simulink model "ZPTEC_state_feedback"  (R2020b)
settings: Solver=FixedStepAuto  StartTime=0.0  StopTime=1  FixedStep=0.002  RelTol=1e-3  EnableMultiTasking=on
values from neighbouring files (symbols this model uses):
  A = [0 1 ... (first row only)    [TestDIST_EFFECT_DCmotor_zp(1).m]    (also in TestDIST_EFFECT_DCmotor_zp.m; lqr_DOB_2_5.mat = [0  1; 0  0]; lqr_DOB_5.mat = [0  1; 0  0]; lqr_DOB_8.mat = [0  1; 0  0])
  B = [0; Kt/Rm/Jt]    [TestDIST_EFFECT_DCmotor_zp(1).m]    (also in TestDIST_EFFECT_DCmotor_zp.m; lqr_DOB_2_5.mat = [0 239.250934036]; lqr_DOB_5.mat = [0 239.250934036]; lqr_DOB_8.mat = [0 239.250934036])
  d = [1 -1.75526480336 0.782027160212]    [lqr_DOB_2_5.mat]    (also in lqr_DOB_5.mat; lqr_DOB_8.mat; lqr_noDOB_10.mat = [1 -1.7546251878 0.781376862182]; lqr_noDOB_2_5.mat = [1 -1.7546251878 0.781376862182])
  K = KK    [TestDIST_EFFECT_DCmotor_zp.m]    (also in lqr_DOB_2_5.mat = [27.9647466006 0.483496818901]; lqr_DOB_5.mat = [27.9647466006 0.483496818901]; lqr_DOB_8.mat = [27.9647466006 0.483496818901]; lqr_noDOB_10.mat = [28.2374499722 0.447372514694])
  n = n(2:3)    [TestDIST_EFFECT_DCmotor_zp(1).m]    (also in TestDIST_EFFECT_DCmotor_zp.m; lqr_DOB_2_5.mat = [0.0133811834885 0.0133811834885]; lqr_DOB_5.mat = [0.0133811834885 0.0133811834885]; lqr_DOB_8.mat = [0.0133811834885 0.0133811834885])
settings Model: Creator=oboe  LastModifiedBy=Lab-Mec
settings DataIOCC: LimitDataPoints=on  SaveFormat=Array  ReturnWorkspaceOutputs=off
settings OptimizationCC: LifeSpan=inf
settings DebuggingCC: SolverPrmCheckMsg=warning  SFUnexpectedBacktrackingDiag=warning  SFNoUnconditionalDefaultTransitionDiag=warning  SFExecutionAtInitializationDiag=none  ArithmeticOperatorsInVariantConditions=warning
settings HardwareCC: ProdBitPerPointer=32  ProdBitPerSizeT=32  ProdBitPerPtrDiffT=32  ProdLargestAtomicFloat=None  ProdIntDivRoundTo=Undefined  ProdEndianess=Unspecified  ProdWordSize=32  ProdHWDeviceType=32-bit Generic
settings ModelReferenceCC: PropagateSignalLabelsOutOfModel=off
settings SFSimCC: SimUseLocalCustomCode=off  CustomCodeUndefinedFunction=UseInterfaceOnly
settings RTWCC: RTWUseLocalCustomCode=off
settings CodeAppCC: StateflowObjectComments=on
settings GRTTargetCC: TargetLangStandard=C89/C90 (ANSI)
settings ConfigComp: CovMetricSettings=dw  CovSaveCumulativeToWorkspaceVar=on  CovSaveSingleToWorkspaceVar=on  CovExternalEMLEnable=off  CovSFcnEnable=off

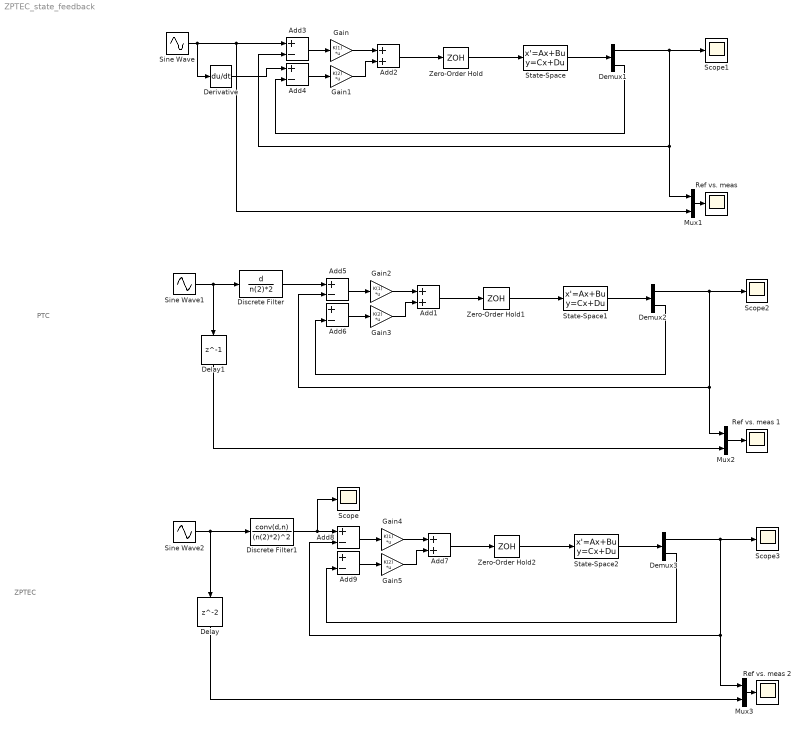
== system ZPTEC_state_feedback ==
  note: PTC
  note: ZPTEC
  Add1 : Sum
  Add2 : Sum
  Add{3..6,8..9} (6 alike) : Sum  Inputs=+-
  Add7 : Sum
  Delay : Delay
  Delay1 : Delay  DelayLength=1
  Demux1 : Demux  Outputs=2
  Demux2 : Demux  Outputs=2
  Demux3 : Demux  Outputs=2
  Derivative : Derivative
  Discrete Filter : DiscreteFilter  Numerator=d  Denominator=n(2)*2  SampleTime=.002
  Discrete Filter1 : DiscreteFilter  Numerator=conv(d,n)  Denominator=(n(2)*2)^2  SampleTime=.002
  Gain : Gain  Gain=K(1)  Multiplication=Matrix(K*u)
  Gain1 : Gain  Gain=K(2)  Multiplication=Matrix(K*u)
  Gain2 : Gain  Gain=K(1)  Multiplication=Matrix(K*u)
  Gain3 : Gain  Gain=K(2)  Multiplication=Matrix(K*u)
  Gain4 : Gain  Gain=K(1)  Multiplication=Matrix(K*u)
  Gain5 : Gain  Gain=K(2)  Multiplication=Matrix(K*u)
  Mux1 : Mux  Inputs=2
  Mux2 : Mux  Inputs=2
  Mux3 : Mux  Inputs=2
  Ref vs. meas : Scope
  Ref vs. meas 1 : Scope
  "Ref vs. meas 2 " : Scope
  Scope{,1..3} (4 alike) : Scope
  Sine Wave : Sin  SineType=Sample based  Amplitude=0.1  Samples=50  SampleTime=.002
  Sine Wave1 : Sin  SineType=Sample based  Amplitude=0.1  Samples=50  SampleTime=.002
  Sine Wave2 : Sin  SineType=Sample based  Amplitude=0.1  Samples=50  SampleTime=.002
  State-Space : StateSpace  A=A(1:2,1:2)  B=B(1:2)  C=eye(2)  D=[0;0]  InitialCondition=0
  State-Space1 : StateSpace  A=A(1:2,1:2)  B=B(1:2)  C=eye(2)  D=[0;0]  InitialCondition=0
  State-Space2 : StateSpace  A=A(1:2,1:2)  B=B(1:2)  C=eye(2)  D=[0;0]  InitialCondition=0
  Zero-Order Hold : ZeroOrderHold  SampleTime=0.002
  Zero-Order Hold1 : ZeroOrderHold  SampleTime=0.002
  Zero-Order Hold2 : ZeroOrderHold  SampleTime=0.002
  wires:
  Mux1/1 -> Ref vs. meas/1
  Zero-Order Hold/1 -> State-Space/1
  Demux1/1 -> Add3/2, Mux1/1, Scope1/1
  Gain/1 -> Add2/1
  Add2/1 -> Zero-Order Hold/1
  Gain1/1 -> Add2/2
  State-Space/1 -> Demux1/1
  Sine Wave/1 -> Mux1/2, Add3/1, Derivative/1
  Demux1/2 -> Add4/2
  Add4/1 -> Gain1/1
  Add3/1 -> Gain/1
  Mux2/1 -> Ref vs. meas 1/1
  Zero-Order Hold1/1 -> State-Space1/1
  Demux2/1 -> Add5/2, Mux2/1, Scope2/1
  Gain2/1 -> Add1/1
  Add1/1 -> Zero-Order Hold1/1
  Gain3/1 -> Add1/2
  State-Space1/1 -> Demux2/1
  Sine Wave1/1 -> Discrete Filter/1, Delay1/1
  Demux2/2 -> Add6/2
  Add6/1 -> Gain3/1
  Add5/1 -> Gain2/1
  Mux3/1 -> "Ref vs. meas 2 "/1
  Zero-Order Hold2/1 -> State-Space2/1
  Demux3/1 -> Add8/2, Mux3/1, Scope3/1
  Gain4/1 -> Add7/1
  Add7/1 -> Zero-Order Hold2/1
  Gain5/1 -> Add7/2
  State-Space2/1 -> Demux3/1
  Demux3/2 -> Add9/2
  Add9/1 -> Gain5/1
  Add8/1 -> Gain4/1
  Delay/1 -> Mux3/2
  Delay1/1 -> Mux2/2
  Discrete Filter1/1 -> Scope/1, Add8/1
  Sine Wave2/1 -> Discrete Filter1/1, Delay/1
  Discrete Filter/1 -> Add5/1
  Derivative/1 -> Add4/1
